simulink subsystem "LinInversePendulum"  (R2023a)
settings: Solver=VariableStepAuto  StartTime=0.0  StopTime=10.0  RelTol=1e-3
values from neighbouring files (symbols this model uses):
  A = [0,     1,                  0,       0 ... (first row only)    [constants.m]
  B = [0;     (m*l^2 + J)/Cv;    0;    -m*l/Cv]    [constants.m]
  C = [0 0 1 0]    [constants.m]
undefined symbols (not defined in the file or in its folder): x0
settings Model: Creator=ycheb  LastModifiedBy=Edgar

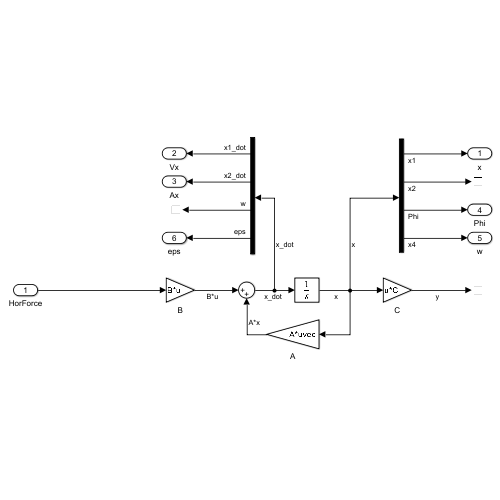
[thumbnail: Simulink's stored preview of the top-level diagram]
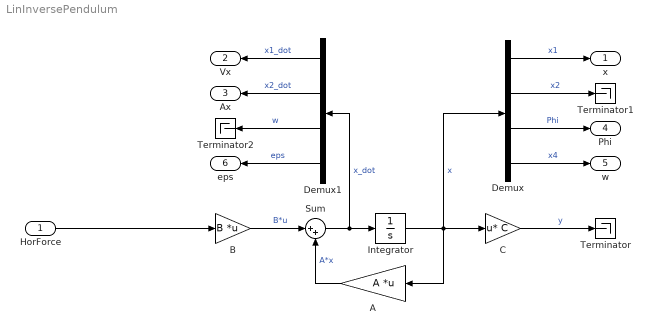
== system LinInversePendulum ==
  HorForce : Inport
  A : Gain  Gain=A  Multiplication=Matrix(K*u) (u vector)
  B : Gain  Gain=B  Multiplication=Matrix(K*u)
  C : Gain  Gain=C  Multiplication=Matrix(u*K)
  Demux : Demux
  Demux1 : Demux
  Integrator : Integrator  InitialCondition=x0
  Sum : Sum  Inputs=|++
  Terminator : Terminator
  Terminator1 : Terminator
  Terminator2 : Terminator
  x : Outport
  Vx : Outport  Port=2
  Ax : Outport  Port=3
  Phi : Outport  Port=4
  w : Outport  Port=5
  eps : Outport  Port=6
  wires:
  Demux/1 -> x/1  "x1"
  Demux1/4 -> eps/1  "eps"
  Demux1/1 -> Vx/1  "x1_dot"
  Demux1/2 -> Ax/1  "x2_dot"
  Demux/3 -> Phi/1  "Phi"
  Demux/4 -> w/1  "x4"
  C/1 -> Terminator/1  "y"
  A/1 -> Sum/2  "A*x"
  Sum/1 -> Integrator/1, Demux1/1  "x_dot"
  HorForce/1 -> B/1
  B/1 -> Sum/1  "B*u"
  Integrator/1 -> A/1, Demux/1, C/1  "x"
  Demux/2 -> Terminator1/1  "x2"
  Demux1/3 -> Terminator2/1  "w"
